simulink model "model_2_Voltage_controlled_single_phase_induction_motor"  (R2023b)
settings: Solver=VariableStepAuto  StartTime=0.0  StopTime=10.0  MaxStep=1e-4  RelTol=1e-3
undefined symbols (not defined in the file): Capacitor, Start
libraries: spsSinglePhaseAsynchronousMachineLib x2, spsACVoltageSourceLib x1, spsControlledVoltageSourceLib x1, simulink x1, spsVoltageMeasurementLib x1, sps_lib x1, spspowerguiLib x1
settings Model: Creator=Haier  LastModifiedBy=Haier

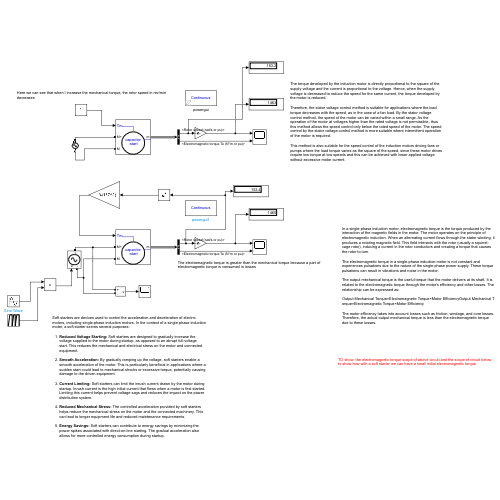
[thumbnail: Simulink's stored preview of the top-level diagram]
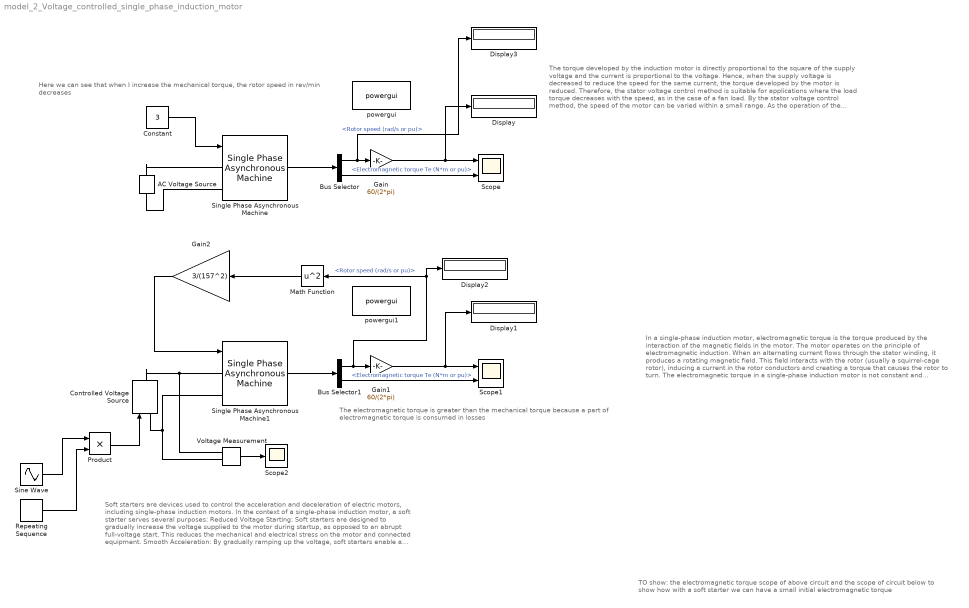
== system model_2_Voltage_controlled_single_phase_induction_motor ==
  note: TO show: the electromagnetic torque scope of above circuit and the scope of circuit below to show how with a soft starter we can have a small initial electromagnetic torque
  note: The electromagnetic torque is greater than the mechanical torque because a part of electromagnetic torque is consumed in losses
  note: In a single-phase induction motor, electromagnetic torque is the torque produced by the interaction of the magnetic fields in the motor. The motor operates on the principle of electromagnetic induction. When an alternating current flows through the stator winding, it produces a rotating magnetic field. This field interacts with the rotor (usually a squirrel-cage rotor), inducing a current in the rotor conductors and creating a torque that causes the rotor to turn.
      | The electromagnetic torque in a single-phase induction motor is not constant and experiences pulsations due to the nature of the single-phase power supply. These torque pulsations can result in vibrations and noise in the motor.
      | The output mechanical torque is the useful torque that the motor delivers at its shaft. It is related to the electromagnetic torque through the motor's efficiency and other losses. The relationship can be expressed as:
      | Output Mechanical Torque=Electromagnetic Torque×Motor EfficiencyOutput Mechanical Torque=Electromagnetic Torque×Motor Efficiency
      | The motor efficiency takes into account losses such as friction, windage, and core losses. Therefore, the actual output mechanical torque is less than the electromagnetic torque due to these losses.
  note: Soft starters are devices used to control the acceleration and deceleration of electric motors, including single-phase induction motors. In the context of a single-phase induction motor, a soft starter serves several purposes:
      | Reduced Voltage Starting: Soft starters are designed to gradually increase the voltage supplied to the motor during startup, as opposed to an abrupt full-voltage start. This reduces the mechanical and electrical stress on the motor and connected equipment.
      | Smooth Acceleration: By gradually ramping up the voltage, soft starters enable a smooth acceleration of the motor. This is particularly beneficial in applications where a sudden start could lead to mechanical shocks or excessive torque, potentially causing damage to the driven equipment.
      | Current Limiting: Soft starters can limit the inrush current drawn by the motor during startup. Inrush current is the high initial current that flows when a motor is first started. Limiting this current helps prevent voltage sags and reduces the impact on the power distribution system.
      | Reduced Mechanical Stress: The controlled acceleration provided by soft starters helps reduce the mechanical stress on the motor and the connected machinery. This can lead to longer equipment life and reduced maintenance requirements.
      | Energy Savings: Soft starters can contribute to energy savings by minimizing the power spikes associated with direct-on-line starting. The gradual acceleration also allows for more controlled energy consumption during startup.
  note: Here we can see that when I increase the mechanical torque, the rotor speed in rev/min decreases
  note: The torque developed by the induction motor is directly proportional to the square of the supply voltage and the current is proportional to the voltage. Hence, when the supply voltage is decreased to reduce the speed for the same current, the torque developed by the motor is reduced.
      |
      | Therefore, the stator voltage control method is suitable for applications where the load torque decreases with the speed, as in the case of a fan load. By the stator voltage control method, the speed of the motor can be varied within a small range. As the operation of the motor at voltages higher than the rated voltage is not permissible, thus this method allows the speed control only below the rated speed of the motor. The speed control by the stator voltage control method is more suitable where intermittent operation of the motor is required.
      |
      | This method is also suitable for the speed control of the induction motors driving fans or pumps where the load torque varies as the square of the speed, since these motor drives require low torque at low speeds and this can be achieved with lower applied voltage without excessive motor current.
  AC Voltage Source : spsACVoltageSourceLib/AC Voltage Source  Amplitude=220*(sqrt(2))  Phase=0  Frequency=50  SampleTime=0  Measurements=None  BusType=swing  Pref=10e3  Qref=0  Qmin=-inf  Qmax=+inf
  Bus Selector : BusSelector  OutputSignals=Mechanical.Rotor speed (rad/s or pu),Mechanical.Electromagnetic torque Te (N*m or pu)
  Bus Selector1 : BusSelector  OutputSignals=Mechanical.Rotor speed (rad/s or pu),Mechanical.Electromagnetic torque Te (N*m or pu)
  Constant : Constant  Value=3
  Controlled Voltage Source : spsControlledVoltageSourceLib/Controlled Voltage Source  Initialize=on  Source_Type=AC  Amplitude=0  Phase=0  Frequency=0  Measurements=None
  Display{,1..3} (4 alike) : Display
  Gain : Gain  Gain=60/(2*pi)
  Gain1 : Gain  Gain=60/(2*pi)
  Gain2 : Gain  Gain=3/(157^2)
  Math Function : Math  Operator=square
  Product : Product
  Repeating Sequence : simulink/Sources/Repeating Sequence  rep_seq_t=[0 4 10]  rep_seq_y=[0 1 1]
  Scope : Scope  NumInputPorts=2
  Scope1 : Scope  NumInputPorts=2
  Scope2 : Scope
  Sine Wave : Sin  Amplitude=220*(sqrt(2))  Frequency=100*pi  SampleTime=0
  Single Phase Asynchronous Machine : spsSinglePhaseAsynchronousMachineLib/Single Phase Asynchronous Machine  MechanicalLoad=Torque Tm  UNITS=SI  MachineType=Capacitor-Start  MeasurementBus=off  NominalParameters="[ .25*746  220  50]"  MainWindingStator="[2.02  7.4e-3]"  MainWindingRotor="[4.12  5.6e-3]"  MutualInductance=0.1772  AuxiliaryWinding="[7.14  8.5e-3]"  Mechanical="[0.0146  0  2 1.18]"  CapacitorStart="[2  254.7e-6]"  CapacitorRun="[18  21.1e-6]"  DisconnectionSpeed=75  InitialSpeed=0  DataType=SI  TsPowergui=0  TsBlock=-1
      settings: LibrarySourceBlock=|
      | sps_lib/Electrical Machines/Single Phase
      | Asynchronous Machine
  Single Phase Asynchronous Machine1 : spsSinglePhaseAsynchronousMachineLib/Single Phase Asynchronous Machine  MechanicalLoad=Torque Tm  UNITS=SI  MachineType=Capacitor-Start  MeasurementBus=off  NominalParameters="[ .25*746  220  50]"  MainWindingStator="[2.02  7.4e-3]"  MainWindingRotor="[4.12  5.6e-3]"  MutualInductance=0.1772  AuxiliaryWinding="[7.14  8.5e-3]"  Mechanical="[0.0146  0  2 1.18]"  CapacitorStart="[2  254.7e-6]"  CapacitorRun="[18  21.1e-6]"  DisconnectionSpeed=75  InitialSpeed=0  DataType=SI  TsPowergui=0  TsBlock=-1
      settings: LibrarySourceBlock=|
      | sps_lib/Electrical Machines/Single Phase
      | Asynchronous Machine
  Voltage Measurement : spsVoltageMeasurementLib/Voltage Measurement  PhasorSimulation=off  OutputType=Complex  PSBequivalent=0
  powergui : sps_lib/powergui  Priority=1  SimulationMode=Continuous  SampleTime=50e-6  frequency=60  Iterations=50  frequencyindice=50  Pbase=100e6  ErrMax=1e-4  UnitsV=kV  UnitsW=MW  buscounter=0  FunctionMessages=off  echomessages=off  EnableUseOfTLC=off  CurrentSourceSwitches=off  DisableSnubberDevices=off  DisableRonSwitches=off  DisableVfSwitches=off  DisplayEquations=off  AutomaticDiscreteSolvers=off  SolverType=Tustin/Backward Euler (TBE)  Interpol=off  ExternalGateDelay=off  methode=off  Ts=100  x0status=blocks  SPID=on  SwTol=0  HookPort=off  NonlinearTolerance=1e-4  nMaxIteration=100  ContinueOnMaxIteration=off  RestoreLinks=warning  ResistiveCurrentMeasurement=off  Frange=[0:2:500]  Ylog=off  Xlog=on  ShowGrid=off  save=off  variable=ZData  structure=0  ZoomFFT=off  StartTime=0.0  cycles=1  DisplayStyle=1  fundamental=60  FreqAxis=off  MaxFrequency=1000  frequencyindicesteady=1  RmsSteady=1  display=off
  powergui1 : spspowerguiLib/powergui  Priority=1  SimulationMode=Continuous  SampleTime=50e-6  frequency=60  Iterations=50  frequencyindice=50  Pbase=100e6  ErrMax=1e-4  UnitsV=kV  UnitsW=MW  buscounter=0  FunctionMessages=off  echomessages=off  EnableUseOfTLC=off  CurrentSourceSwitches=off  DisableSnubberDevices=off  DisableRonSwitches=off  DisableVfSwitches=off  DisplayEquations=off  AutomaticDiscreteSolvers=off  SolverType=Tustin/Backward Euler (TBE)  Interpol=off  ExternalGateDelay=off  methode=off  Ts=100  x0status=blocks  SPID=on  SwTol=0  HookPort=off  NonlinearTolerance=1e-4  nMaxIteration=100  ContinueOnMaxIteration=off  RestoreLinks=warning  ResistiveCurrentMeasurement=off  Frange=[0:2:500]  Ylog=off  Xlog=on  ShowGrid=off  save=off  variable=ZData  structure=0  ZoomFFT=off  StartTime=0.0  cycles=1  DisplayStyle=1  fundamental=60  FreqAxis=off  MaxFrequency=1000  frequencyindicesteady=1  RmsSteady=1  display=off
  wires:
  Single Phase Asynchronous Machine/1 -> Bus Selector/1
  Constant/1 -> Single Phase Asynchronous Machine/1
  Bus Selector/1 -> Display3/1, Gain/1  "<Rotor speed (rad/s or pu)>"
  Bus Selector/2 -> Scope/2  "<Electromagnetic torque Te (N*m or pu)>"
  Gain/1 -> Display/1, Scope/1
  Single Phase Asynchronous Machine1/1 -> Bus Selector1/1
  Bus Selector1/1 -> Math Function/1, Display2/1, Gain1/1  "<Rotor speed (rad/s or pu)>"
  Gain1/1 -> Display1/1, Scope1/1
  Bus Selector1/2 -> Scope1/2  "<Electromagnetic torque Te (N*m or pu)>"
  Gain2/1 -> Single Phase Asynchronous Machine1/1
  Math Function/1 -> Gain2/1
  Voltage Measurement/1 -> Scope2/1
  Product/1 -> Controlled Voltage Source/1
  Sine Wave/1 -> Product/1
  Repeating Sequence/1 -> Product/2
  connections:
  AC Voltage Source/RConn1 -- Single Phase Asynchronous Machine/LConn1
  AC Voltage Source/LConn1 -- Single Phase Asynchronous Machine/LConn2
  Controlled Voltage Source/RConn1 -- Voltage Measurement/LConn1 -- Single Phase Asynchronous Machine1/LConn1
  Single Phase Asynchronous Machine1/LConn2 -- Voltage Measurement/LConn2 -- Controlled Voltage Source/LConn1
